simulink model "moving_car"  (R2018b)
settings: Solver=VariableStepAuto  StartTime=0.0  StopTime=10.0  RelTol=1e-3
libraries: simulink x1
settings Model: Creator=obas  LastModifiedBy=Lenovo
settings SolverCC: DecoupledContinuousIntegration=on  MinimalZcImpactIntegration=on
settings DebuggingCC: LibraryContextMissingDiagnostic=none
settings SFSimCC: SimUseLocalCustomCode=off
settings RTWCC: RTWUseLocalCustomCode=off

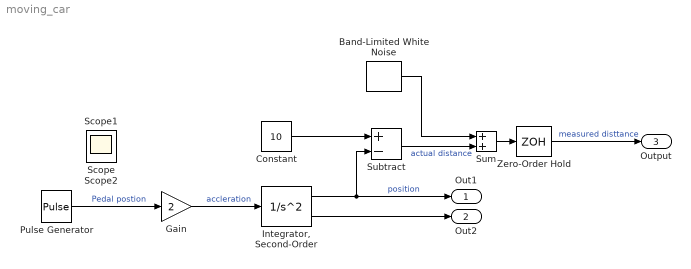
== system moving_car ==
  Band-Limited White Noise : simulink/Sources/Band-Limited White Noise  Cov=0.001  Ts=0.1  seed=[23341]
  Constant : Constant  Value=10
  Gain : Gain  Gain=2
  "Integrator, Second-Order" : SecondOrderIntegrator  LimitX=on  UpperLimitX=10
  Pulse Generator : DiscretePulseGenerator  PulseType=Time based  Period=10  PulseWidth=5
  Subtract : Sum  Inputs=+-
  Sum : Sum
  Zero-Order Hold : ZeroOrderHold  SampleTime=0.1
  Out1 : Outport
  Out2 : Outport  Port=2
  Output : Outport  Port=3
  Scope : Scope
  Scope1 : Scope
  Scope2 : Scope
  wires:
  "Integrator, Second-Order"/1 -> Subtract/2, Out1/1  "position"
  "Integrator, Second-Order"/2 -> Out2/1
  Gain/1 -> "Integrator, Second-Order"/1  "accleration"
  Pulse Generator/1 -> Gain/1  "Pedal postion"
  Constant/1 -> Subtract/1
  Band-Limited White Noise/1 -> Sum/1
  Subtract/1 -> Sum/2  "actual distance"
  Sum/1 -> Zero-Order Hold/1
  Zero-Order Hold/1 -> Output/1  "measured disttance"
